simulink model "schemi_simulink"  (R2020a)
settings: Solver=VariableStepAuto  StartTime=0.0  StopTime=30  RelTol=1e-3
values from neighbouring files (symbols this model uses):
  A = [-m-a*y1/x_max+2*m*x1/x_max    a-a*x1/x_max;      b-b*y1/y_max  -n-b*x1/y_max+2*n*y1/y_max]    [linearized.m]
  A1 = [-m1-a1*y1/x_max1+2*m1*x1/x_max    a-a*x1/x_max1;      b1-b1*y1/y_max  -n1-b1*x1/y_max+2*n1*y1/y_max1]    [linearized.m]
  B = [1-x1/x_max;1-y1/y_max]    [linearized.m]
  B1 = [1-x1/x_max1;1-y1/y_max1]    [linearized.m]
  C = [1 0]    [linearized.m]
  D = 0    [linearized.m]
  dis = -0.3    [linearized.m]    (also in main.m = 0.3)
  Kf = KK(:,1:2)    [linearized.m]
  Kfm = KKm(:,1:2)    [linearized.m]
  Ki = KK(:,end)    [linearized.m]
  Kim = KKm(:,end)    [linearized.m]
  rif = 1    [linearized.m]    (also in main.m)
  td = 10    [linearized.m]
  x_ini = [0.1;0.1]    [linearized.m]
libraries: simulink x3
settings Model: Creator=ThinkPad  LastModifiedBy=ThinkPad

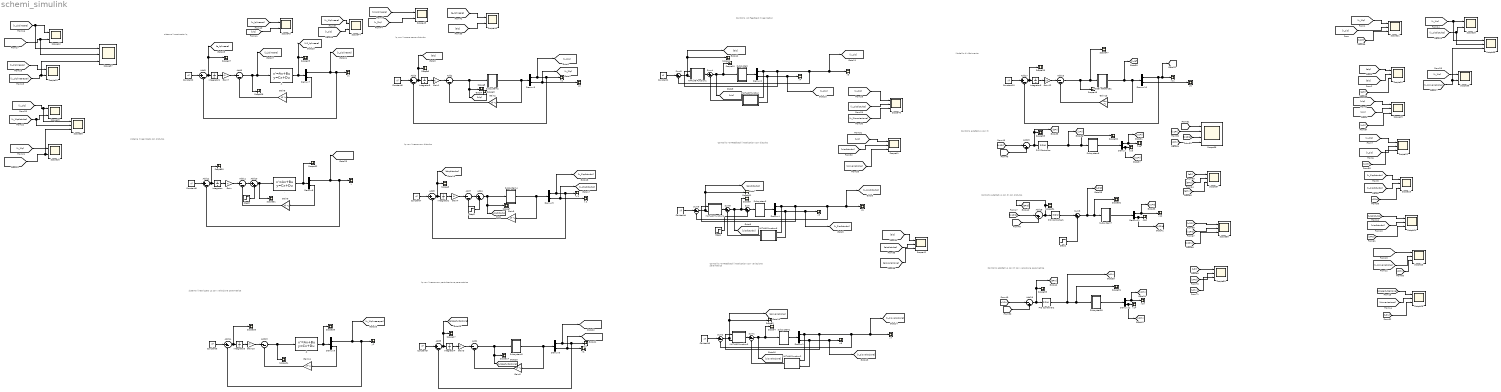
== system schemi_simulink ==
  note: Modello di riferimento
  note: Controllo I-O Feedback linearization
  note: Controllo I-O Feedback linearization con variazione parametrica
  note: Controllo I-O Feedback linearization con disturbo
  note: lq non lineare senza disturbo
  note: lq non lineare con disturbo
  note: lq non lineare con perturbazione parametrica
  note: sistema linearizzato lq
  note: sistema linearizzato con disturbo
  note: sistema linearizzato Lq con variazione parametrica
  note: Controllo adattativo con PI con disturbo
  note: Controllo adattativo con PI con variazione parametrica
  note: Controllo adattativo con PI
  . : StateSpace  A=A  B=B  C=[C; eye(2)]  D=[D; zeros(2,1)]  InitialCondition=x_ini
  .1 : StateSpace  A=A  B=B  C=[C; eye(2)]  D=[D; zeros(2,1)]  InitialCondition=x_ini
  .2 : StateSpace  A=A1  B=B1  C=[C; eye(2)]  D=[D; zeros(2,1)]  InitialCondition=x_ini
  Add{1..2,6..7,11,13,16} (7 alike) : Sum  Inputs=|--
  Add10 : Sum  Inputs=|++
  Add{3,5,8..9,12,14,17} (7 alike) : Sum  Inputs=|+-
  Add15 : Sum  Inputs=|-+
  Add18 : Sum  Inputs=|-+
  Add19 : Sum  Inputs=|-+
  Add4 : Sum  Inputs=|++
  Constant{1..10} (10 alike) : Constant  Value=rif
  Demux : Demux  Outputs=2
  Demux{1..6,10} (7 alike) : Demux  Outputs=[1 1]
  Demux11 : Demux  Outputs=2
  Demux12 : Demux  Outputs=2
  Demux7 : Demux  Outputs=[1 2]
  Demux8 : Demux  Outputs=[1 2]
  Demux9 : Demux  Outputs=[1 2]
  Gain{,1,3..4,7,10} (6 alike) : Gain  Gain=Ki
  Gain{2,5..6,8..9,11} (6 alike) : Gain  Gain=Kf  Multiplication=Matrix(K*u)
  Gain12 : Gain  Gain=Kim
  Gain13 : Gain  Gain=Kfm  Multiplication=Matrix(K*u)
  Integrator{,1..6} (7 alike) : Integrator
  MATLAB Function : MATLAB Function  TreatAsAtomicUnit=on
  MATLAB Function1 : MATLAB Function  TreatAsAtomicUnit=on
  MATLAB Function2 : MATLAB Function  TreatAsAtomicUnit=on
  MATLAB Function3 : MATLAB Function  TreatAsAtomicUnit=on
  MATLAB Function4 : MATLAB Function  TreatAsAtomicUnit=on
  MATLAB Function6 : MATLAB Function  TreatAsAtomicUnit=on
  Model reference1 : Subsystem
  PID Controller : simulink/Continuous/PID Controller  Controller=PID  Form=Parallel  TimeDomain=Continuous-time  UseExternalTs=off  SampleTime=-1  IntegratorMethod=Forward Euler  FilterMethod=Forward Euler  ControllerParametersSource=internal  P=10  I=20  D=0  UseFilter=on  N=100  TunerSelectOption=Transfer Function Based (PID Tuner App)  InitialConditionSource=internal  InitialConditionForIntegrator=0  InitialConditionForFilter=0  DifferentiatorICPrevScaledInput=0  ExternalReset=none  TrackingMode=off  Kt=1  LimitOutput=off  UpperSaturationLimit=inf  LowerSaturationLimit=-inf  LinearizeAsGain=on  AntiWindupMode=none  Kb=1  POutMin=[]  POutMax=[]  IOutMin=[]  IOutMax=[]  DOutMin=[]  DOutMax=[]  NOutMin=[]  NOutMax=[]  SumOutMin=[]  SumOutMax=[]  SaturationOutMin=[]  SaturationOutMax=[]  PParamMin=[]  PParamMax=[]  IParamMin=[]  IParamMax=[]  DParamMin=[]  DParamMax=[]  NParamMin=[]  NParamMax=[]  KbParamMin=[]  KbParamMax=[]  KtParamMin=[]  KtParamMax=[]  KbOutMin=[]  KbOutMax=[]  KtOutMin=[]  KtOutMax=[]  IntegratorOutMin=[]  IntegratorOutMax=[]  FilterOutMin=[]  FilterOutMax=[]  SumI1OutMin=[]  SumI1OutMax=[]  SumI2OutMin=[]  SumI2OutMax=[]  SumI3OutMin=[]  SumI3OutMax=[]  SumI4OutMin=[]  SumI4OutMax=[]  SumDOutMin=[]  SumDOutMax=[]  DifferentiatorOutMin=[]  DifferentiatorOutMax=[]  FilterDiffOutCoefMin=[]  FilterDiffOutCoefMax=[]  ReciprocalOutMin=[]  ReciprocalOutMax=[]  SumDenOutMin=[]  SumDenOutMax=[]  SumNumOutMin=[]  SumNumOutMax=[]  DivideOutMin=[]  DivideOutMax=[]  UdiffTsProdOutMin=[]  UdiffTsProdOutMax=[]  NTsProdOutMin=[]  NTsProdOutMax=[]  UintegralTsProdOutMin=[]  UintegralTsProdOutMax=[]  UngainTsProdOutMin=[]  UngainTsProdOutMax=[]  IntegratorContinuousStateAttributes=''  IntegratorStateMustResolveToSignalObject=off  IntegratorRTWStateStorageClass=Auto  FilterContinuousStateAttributes=''  FilterStateMustResolveToSignalObject=off  FilterRTWStateStorageClass=Auto  ParallelPVariant=InternalParameters  IdealPVariant=Disabled  IVariant=InternalParameters  DVariant=InternalParameters  IntegratorVariant=Continuous  SatVariant=Disabled  AWVariant=Passthrough  PCopyVariant=Disabled  TRVariant=Disabled  FdbkBlocksVariant=Forward  IdealPFdbkVariant=Disabled  SatFdbkVariant=Disabled  DerivativeFilterVariant=ContFilter  NVariant=InternalParameters  NCopyVariant=Disabled  FilterICVariant=InternalICsFilter  IntegratorICVariant=InternalICs  ExternalResetVariant=Disabled  TRSumVariant=Passthrough  SumFdbkVariant=Disabled  SumVariant=Sum_PID  TsampFilterVariant=InternalTs  TsampNgainVariant=Passthrough  TsampIntegralVariant=Passthrough
  PID Controller1 : simulink/Continuous/PID Controller  Controller=PID  Form=Parallel  TimeDomain=Continuous-time  UseExternalTs=off  SampleTime=-1  IntegratorMethod=Forward Euler  FilterMethod=Forward Euler  ControllerParametersSource=internal  P=10  I=20  D=0  UseFilter=on  N=100  TunerSelectOption=Transfer Function Based (PID Tuner App)  InitialConditionSource=internal  InitialConditionForIntegrator=0  InitialConditionForFilter=0  DifferentiatorICPrevScaledInput=0  ExternalReset=none  TrackingMode=off  Kt=1  LimitOutput=off  UpperSaturationLimit=inf  LowerSaturationLimit=-inf  LinearizeAsGain=on  AntiWindupMode=none  Kb=1  POutMin=[]  POutMax=[]  IOutMin=[]  IOutMax=[]  DOutMin=[]  DOutMax=[]  NOutMin=[]  NOutMax=[]  SumOutMin=[]  SumOutMax=[]  SaturationOutMin=[]  SaturationOutMax=[]  PParamMin=[]  PParamMax=[]  IParamMin=[]  IParamMax=[]  DParamMin=[]  DParamMax=[]  NParamMin=[]  NParamMax=[]  KbParamMin=[]  KbParamMax=[]  KtParamMin=[]  KtParamMax=[]  KbOutMin=[]  KbOutMax=[]  KtOutMin=[]  KtOutMax=[]  IntegratorOutMin=[]  IntegratorOutMax=[]  FilterOutMin=[]  FilterOutMax=[]  SumI1OutMin=[]  SumI1OutMax=[]  SumI2OutMin=[]  SumI2OutMax=[]  SumI3OutMin=[]  SumI3OutMax=[]  SumI4OutMin=[]  SumI4OutMax=[]  SumDOutMin=[]  SumDOutMax=[]  DifferentiatorOutMin=[]  DifferentiatorOutMax=[]  FilterDiffOutCoefMin=[]  FilterDiffOutCoefMax=[]  ReciprocalOutMin=[]  ReciprocalOutMax=[]  SumDenOutMin=[]  SumDenOutMax=[]  SumNumOutMin=[]  SumNumOutMax=[]  DivideOutMin=[]  DivideOutMax=[]  UdiffTsProdOutMin=[]  UdiffTsProdOutMax=[]  NTsProdOutMin=[]  NTsProdOutMax=[]  UintegralTsProdOutMin=[]  UintegralTsProdOutMax=[]  UngainTsProdOutMin=[]  UngainTsProdOutMax=[]  IntegratorContinuousStateAttributes=''  IntegratorStateMustResolveToSignalObject=off  IntegratorRTWStateStorageClass=Auto  FilterContinuousStateAttributes=''  FilterStateMustResolveToSignalObject=off  FilterRTWStateStorageClass=Auto  ParallelPVariant=InternalParameters  IdealPVariant=Disabled  IVariant=InternalParameters  DVariant=InternalParameters  IntegratorVariant=Continuous  SatVariant=Disabled  AWVariant=Passthrough  PCopyVariant=Disabled  TRVariant=Disabled  FdbkBlocksVariant=Forward  IdealPFdbkVariant=Disabled  SatFdbkVariant=Disabled  DerivativeFilterVariant=ContFilter  NVariant=InternalParameters  NCopyVariant=Disabled  FilterICVariant=InternalICsFilter  IntegratorICVariant=InternalICs  ExternalResetVariant=Disabled  TRSumVariant=Passthrough  SumFdbkVariant=Disabled  SumVariant=Sum_PID  TsampFilterVariant=InternalTs  TsampNgainVariant=Passthrough  TsampIntegralVariant=Passthrough
  PID Controller2 : simulink/Continuous/PID Controller  Controller=PID  Form=Parallel  TimeDomain=Continuous-time  UseExternalTs=off  SampleTime=-1  IntegratorMethod=Forward Euler  FilterMethod=Forward Euler  ControllerParametersSource=internal  P=10  I=20  D=0  UseFilter=on  N=100  TunerSelectOption=Transfer Function Based (PID Tuner App)  InitialConditionSource=internal  InitialConditionForIntegrator=0  InitialConditionForFilter=0  DifferentiatorICPrevScaledInput=0  ExternalReset=none  TrackingMode=off  Kt=1  LimitOutput=off  UpperSaturationLimit=inf  LowerSaturationLimit=-inf  LinearizeAsGain=on  AntiWindupMode=none  Kb=1  POutMin=[]  POutMax=[]  IOutMin=[]  IOutMax=[]  DOutMin=[]  DOutMax=[]  NOutMin=[]  NOutMax=[]  SumOutMin=[]  SumOutMax=[]  SaturationOutMin=[]  SaturationOutMax=[]  PParamMin=[]  PParamMax=[]  IParamMin=[]  IParamMax=[]  DParamMin=[]  DParamMax=[]  NParamMin=[]  NParamMax=[]  KbParamMin=[]  KbParamMax=[]  KtParamMin=[]  KtParamMax=[]  KbOutMin=[]  KbOutMax=[]  KtOutMin=[]  KtOutMax=[]  IntegratorOutMin=[]  IntegratorOutMax=[]  FilterOutMin=[]  FilterOutMax=[]  SumI1OutMin=[]  SumI1OutMax=[]  SumI2OutMin=[]  SumI2OutMax=[]  SumI3OutMin=[]  SumI3OutMax=[]  SumI4OutMin=[]  SumI4OutMax=[]  SumDOutMin=[]  SumDOutMax=[]  DifferentiatorOutMin=[]  DifferentiatorOutMax=[]  FilterDiffOutCoefMin=[]  FilterDiffOutCoefMax=[]  ReciprocalOutMin=[]  ReciprocalOutMax=[]  SumDenOutMin=[]  SumDenOutMax=[]  SumNumOutMin=[]  SumNumOutMax=[]  DivideOutMin=[]  DivideOutMax=[]  UdiffTsProdOutMin=[]  UdiffTsProdOutMax=[]  NTsProdOutMin=[]  NTsProdOutMax=[]  UintegralTsProdOutMin=[]  UintegralTsProdOutMax=[]  UngainTsProdOutMin=[]  UngainTsProdOutMax=[]  IntegratorContinuousStateAttributes=''  IntegratorStateMustResolveToSignalObject=off  IntegratorRTWStateStorageClass=Auto  FilterContinuousStateAttributes=''  FilterStateMustResolveToSignalObject=off  FilterRTWStateStorageClass=Auto  ParallelPVariant=InternalParameters  IdealPVariant=Disabled  IVariant=InternalParameters  DVariant=InternalParameters  IntegratorVariant=Continuous  SatVariant=Disabled  AWVariant=Passthrough  PCopyVariant=Disabled  TRVariant=Disabled  FdbkBlocksVariant=Forward  IdealPFdbkVariant=Disabled  SatFdbkVariant=Disabled  DerivativeFilterVariant=ContFilter  NVariant=InternalParameters  NCopyVariant=Disabled  FilterICVariant=InternalICsFilter  IntegratorICVariant=InternalICs  ExternalResetVariant=Disabled  TRSumVariant=Passthrough  SumFdbkVariant=Disabled  SumVariant=Sum_PID  TsampFilterVariant=InternalTs  TsampNgainVariant=Passthrough  TsampIntegralVariant=Passthrough
  Scope{1..11,14,17,27..35,47..55} (31 alike) : Scope
  Scope{12..13,15..16,18,36,43..46} (10 alike) : Scope  NumInputPorts=2
  Scope{19..26,37..42,57..59} (17 alike) : Scope  NumInputPorts=3
  Scope56 : Scope  NumInputPorts=4
  Step{1..2,5,8} (4 alike) : Step  Time=td  After=dis  SampleTime=0
  Subsystem : Subsystem
  Subsystem1 : Subsystem
  Subsystem2 : Subsystem
  Subsystem3 : Subsystem
  Subsystem4 : Subsystem
  Subsystem5 : Subsystem
  Subsystem6 : Subsystem
  Subsystem7 : Subsystem
  Subsystem9 : Subsystem
  Sum : Sum  Inputs=|++
  Sum{1..2,4..5,8..9} (6 alike) : Sum  Inputs=|+-
  Sum3 : Sum  Inputs=|++
  x.1 : Scope
  x.2 : Scope
  x{1..16} (16 alike) : Scope
  x1. : Scope
  x2. : Scope
  y : Scope
  y1 : Scope
  y2 : Scope
  wires:
  MATLAB Function/1(y) -> Sum4/2
  Constant1/1 -> Sum5/1
  Subsystem/1(Out1) -> Demux2/1
  MATLAB Function1/1(y) -> Sum4/1
  Sum5/1 -> [eio], Scope1/1, MATLAB Function1/2(e)  "e"
  Demux2/1 -> MATLAB Function/1(x_1), x3/1, [x_1io], Sum5/2, MATLAB Function1/1(x_1)
  Demux2/2 -> MATLAB Function/2(x_2), x4/1, [x_2io]
  Sum4/1 -> [uio], Scope10/1, Subsystem/1(u)  "u"
  Subsystem3/1(Out1) -> Demux4/1
  Demux4/2 -> MATLAB Function6/2(x_2), x5/1, [x_2iodisturbo]
  Demux4/1 -> MATLAB Function6/1(x_1), MATLAB Function4/1(x_1), x6/1, [x_1iodisturbo], Sum9/2
  Sum8/1 -> [uiodisturbo], Scope9/1, Sum/1  "u"
  Sum9/1 -> MATLAB Function4/2(e), Scope11/1, [eiodisturbo]  "e"
  Constant4/1 -> Sum9/1
  MATLAB Function4/1(y) -> Sum8/1
  MATLAB Function6/1(y) -> Sum8/2
  Sum/1 -> Subsystem3/1(u)
  Step1/1 -> Sum/2
  Subsystem1/1(Out1) -> Demux1/1
  Demux1/2 -> MATLAB Function2/2(x_2), x8/1, [x_2iovariazione]
  Demux1/1 -> MATLAB Function2/1(x_1), MATLAB Function3/1(x_1), x7/1, [x_1iovariazione], Sum2/2
  Sum1/1 -> [uiovariazione], Scope4/1, Subsystem1/1(u)  "u"
  Sum2/1 -> MATLAB Function3/2(e), Scope2/1, [eiovariazione]  "e"
  Constant3/1 -> Sum2/1
  MATLAB Function3/1(y) -> Sum1/1
  MATLAB Function2/1(y) -> Sum1/2
  Subsystem2/1(Out1) -> Gain2/1, Demux3/1
  Add2/1 -> [ulq], Scope5/1, Subsystem2/1(u)
  Integrator3/1 -> Gain1/1
  Constant5/1 -> Add3/1
  Demux3/2 -> x2/1, [x_2lq]
  Add3/1 -> Scope6/1, [elq], Integrator3/1
  Demux3/1 -> [x_1lq], x1/1, Add3/2
  Gain1/1 -> Add2/1
  Gain2/1 -> Add2/2
  Add8/1 -> Scope8/1, [elqdisturbo], Integrator2/1
  Constant7/1 -> Add8/1
  Add7/1 -> Add4/1
  Subsystem4/1(Out1) -> Gain5/1, Demux5/1
  Integrator2/1 -> Gain4/1
  Demux5/2 -> [x_2lqdisturbo], x.2/1
  Gain4/1 -> Add7/1
  Demux5/1 -> x.1/1, Add8/2, [x_1lqdisturbo]
  Add4/1 -> Subsystem4/1(u), [ulqdisturbo], Scope7/1
  Step5/1 -> Add4/2
  Gain5/1 -> Add7/2
  Add5/1 -> Scope17/1, [elqperturbazione], Integrator4/1
  Demux6/2 -> x2./1, [x_2lqperturbazione]
  Constant9/1 -> Add5/1
  Subsystem5/1(Out1) -> Gain6/1, Demux6/1
  Gain6/1 -> Add1/2
  Integrator4/1 -> Gain3/1
  Gain3/1 -> Add1/1
  Demux6/1 -> [x_1lqperturbazione], x1./1, Add5/2
  Add1/1 -> Scope14/1, [ulqperturbazione], Subsystem5/1(u)
  [x_1io] -> Scope21/2
  [elq] -> Scope20/1
  [eio] -> Scope20/2
  [ulq] -> Scope19/1
  [uio] -> Scope19/2
  [x_2lq] -> Scope22/1
  [x_2io] -> Scope22/2
  [x_1iodisturbo] -> Scope25/2
  [x_1lqdisturbo] -> Scope25/1
  [ulqdisturbo] -> Scope24/1
  [uiodisturbo] -> Scope24/2
  [uiovariazione] -> Scope26/2
  [ulqperturbazione] -> Scope26/1
  [x_1iovariazione] -> Scope23/2
  [x_1lqperturbazione] -> Scope23/1
  [x_1lq] -> Scope21/1
  Integrator1/1 -> Gain7/1
  Gain7/1 -> Add6/1
  Gain8/1 -> Add6/2
  Demux7/2 -> Gain8/1
  Demux7/1 -> [x_1lqlineare], y1/1, Add9/2
  .1/1 -> [x2_lqlineare], Scope29/1, Demux7/1
  Constant2/1 -> Add9/1
  Gain9/1 -> Add11/2
  Add12/1 -> Scope30/1, Integrator/1
  Gain/1 -> Add11/1
  Step8/1 -> Add10/2
  Add10/1 -> Scope31/1, ./1
  Demux8/2 -> Gain9/1
  Constant8/1 -> Add12/1
  Demux8/1 -> [x_1lqdisturbolineare], y/1, Add12/2
  ./1 -> Scope32/1, Demux8/1
  Integrator/1 -> Gain/1
  Add11/1 -> Add10/1
  Constant6/1 -> Add14/1
  .2/1 -> Scope35/1, Demux9/1
  Add13/1 -> Scope34/1, .2/1
  Demux9/1 -> [x_1lqlineareper], y2/1, Add14/2
  Demux9/2 -> Gain11/1
  Gain11/1 -> Add13/2
  Integrator5/1 -> Gain10/1
  Add14/1 -> Scope33/1, Integrator5/1
  Gain10/1 -> Add13/1
  [x_1lqlineare] -> Scope37/1, Scope12/1
  [x_1lqdisturbolineare] -> Scope37/2, Scope12/2
  [x_1lqlineare] -> Scope13/1
  [x_1lqlineareper] -> Scope37/3, Scope13/2
  [x_1lq] -> Scope38/1, Scope15/1
  [x_1lqdisturbo] -> Scope38/2, Scope15/2
  [x_1lq] -> Scope16/1
  [x_1lqperturbazione] -> Scope38/3, Scope16/2
  [x_1io] -> Scope39/1, Scope18/1
  [x_1iodisturbo] -> Scope39/2, Scope18/2
  [x_1io] -> Scope36/1
  [x_1iovariazione] -> Scope39/3, Scope36/2
  [x_2io] -> Scope40/1
  [x_2iodisturbo] -> Scope40/2
  [x_2iovariazione] -> Scope40/3
  [uio] -> Scope41/1
  [uiodisturbo] -> Scope41/2
  [uiovariazione] -> Scope41/3
  [eio] -> Scope42/1
  [eiodisturbo] -> Scope42/2
  [eiovariazione] -> Scope42/3
  Add6/1 -> Scope28/1, [u_lqlineare], .1/1
  Add9/1 -> [e_lqlineare], Scope27/1, Integrator1/1
  [u_lqlineare] -> Scope43/1
  [ulq] -> Scope43/2
  [x_1lqlineare] -> Scope44/1
  [x_1lq] -> Scope44/2
  [x2_lqlineare] -> Scope45/1
  [x_2lq] -> Scope45/2
  [e_lqlineare] -> Scope46/1
  [elq] -> Scope46/2
  [x1PI] -> Add15/1
  Subsystem6/1(Out1) -> Demux/1
  Add17/1 -> Scope49/1, Integrator6/1
  PID Controller/1 -> [uPI], Scope50/1, Subsystem6/1(u)
  Gain13/1 -> Add16/2
  Demux/2 -> [x2PI], x16/1
  Model reference1/1(Out1) -> [x_ref], Gain13/1, Demux10/1
  Demux10/2 -> x9/1
  Demux/1 -> x13/1, [x1PI]
  [x1_refPI] -> Add15/2
  Add16/1 -> Scope47/1, Model reference1/1(u), Scope48/1
  Demux10/1 -> x11/1, [x1_refPI], Add17/2
  Add15/1 -> [ePI], Scope53/1, PID Controller/1
  Constant10/1 -> Add17/1
  Integrator6/1 -> Gain12/1
  Gain12/1 -> Add16/1
  Add18/1 -> Scope54/1, [ePId], PID Controller1/1
  [x1_refPI] -> Add18/2
  Subsystem7/1(Out1) -> Demux11/1
  Demux11/1 -> [x1PId], x12/1
  [x1PId] -> Add18/1
  Step2/1 -> Sum3/2
  PID Controller1/1 -> Sum3/1
  Sum3/1 -> [uPId], Scope52/1, Subsystem7/1(u)
  Add19/1 -> [ePIv], Scope55/1, PID Controller2/1
  [x1_refPI] -> Add19/2
  Demux12/2 -> [x2PIv], x14/1
  Subsystem9/1(Out1) -> Demux12/1
  PID Controller2/1 -> [uPIv], Scope51/1, Subsystem9/1(u)
  Demux12/1 -> x10/1, [x1PIv]
  [x1PIv] -> Add19/1
  [x1_refPI] -> Scope56/1
  [x1PI] -> Scope56/2
  [x1PId] -> Scope56/3
  [x1PIv] -> Scope56/4
  [x1PI] -> Scope21/3
  [ePI] -> Scope20/3
  [uPI] -> Scope19/3
  [x2PI] -> Scope22/3
  [x1PIv] -> Scope23/3
  [x1PId] -> Scope25/3
  [uPId] -> Scope24/3
  [uPIv] -> Scope26/3
  Demux11/2 -> [x2PId], x15/1
  [ePI] -> Scope57/1
  [ePId] -> Scope57/2
  [ePIv] -> Scope57/3
  [x2PI] -> Scope58/1
  [x2PId] -> Scope58/2
  [x2PIv] -> Scope58/3
  [uPI] -> Scope59/1
  [uPId] -> Scope59/2
  [uPIv] -> Scope59/3

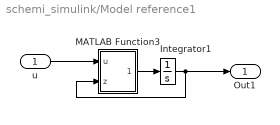
== system schemi_simulink/Model reference1 ==
  u : Inport
  Integrator1 : Integrator  InitialCondition=x_ini
  MATLAB Function3 : MATLAB Function  TreatAsAtomicUnit=on
  Out1 : Outport
  wires:
  u/1 -> MATLAB Function3/1(u)
  MATLAB Function3/1(xi_dot) -> Integrator1/1
  Integrator1/1 -> MATLAB Function3/2(z), Out1/1

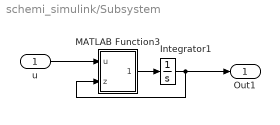
== system schemi_simulink/Subsystem ==
  u : Inport
  Integrator1 : Integrator  InitialCondition=x_ini
  MATLAB Function3 : MATLAB Function  TreatAsAtomicUnit=on
  Out1 : Outport
  wires:
  Integrator1/1 -> Out1/1, MATLAB Function3/2(z)
  MATLAB Function3/1(xi_dot) -> Integrator1/1
  u/1 -> MATLAB Function3/1(u)

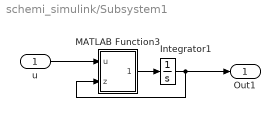
== system schemi_simulink/Subsystem1 ==
  u : Inport
  Integrator1 : Integrator  InitialCondition=x_ini
  MATLAB Function3 : MATLAB Function  TreatAsAtomicUnit=on
  Out1 : Outport
  wires:
  Integrator1/1 -> Out1/1, MATLAB Function3/2(z)
  MATLAB Function3/1(xi_dot) -> Integrator1/1
  u/1 -> MATLAB Function3/1(u)

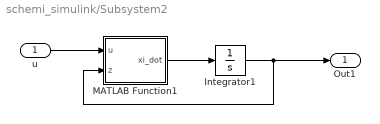
== system schemi_simulink/Subsystem2 ==
  u : Inport
  Integrator1 : Integrator  InitialCondition=x_ini
  MATLAB Function1 : MATLAB Function  TreatAsAtomicUnit=on
  Out1 : Outport
  wires:
  Integrator1/1 -> Out1/1, MATLAB Function1/2(z)
  MATLAB Function1/1(xi_dot) -> Integrator1/1
  u/1 -> MATLAB Function1/1(u)

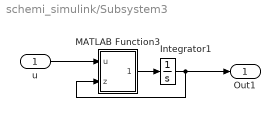
== system schemi_simulink/Subsystem3 ==
  u : Inport
  Integrator1 : Integrator  InitialCondition=x_ini
  MATLAB Function3 : MATLAB Function  TreatAsAtomicUnit=on
  Out1 : Outport
  wires:
  Integrator1/1 -> Out1/1, MATLAB Function3/2(z)
  MATLAB Function3/1(xi_dot) -> Integrator1/1
  u/1 -> MATLAB Function3/1(u)

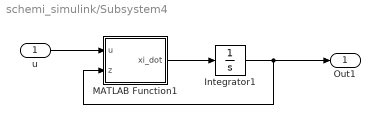
== system schemi_simulink/Subsystem4 ==
  u : Inport
  Integrator1 : Integrator  InitialCondition=x_ini
  MATLAB Function1 : MATLAB Function  TreatAsAtomicUnit=on
  Out1 : Outport
  wires:
  Integrator1/1 -> Out1/1, MATLAB Function1/2(z)
  MATLAB Function1/1(xi_dot) -> Integrator1/1
  u/1 -> MATLAB Function1/1(u)

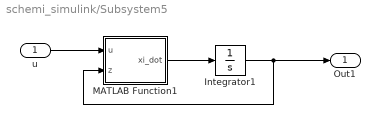
== system schemi_simulink/Subsystem5 ==
  u : Inport
  Integrator1 : Integrator  InitialCondition=x_ini
  MATLAB Function1 : MATLAB Function  TreatAsAtomicUnit=on
  Out1 : Outport
  wires:
  Integrator1/1 -> Out1/1, MATLAB Function1/2(z)
  MATLAB Function1/1(xi_dot) -> Integrator1/1
  u/1 -> MATLAB Function1/1(u)

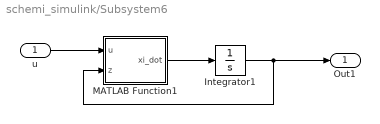
== system schemi_simulink/Subsystem6 ==
  u : Inport
  Integrator1 : Integrator  InitialCondition=x_ini
  MATLAB Function1 : MATLAB Function  TreatAsAtomicUnit=on
  Out1 : Outport
  wires:
  Integrator1/1 -> Out1/1, MATLAB Function1/2(z)
  MATLAB Function1/1(xi_dot) -> Integrator1/1
  u/1 -> MATLAB Function1/1(u)

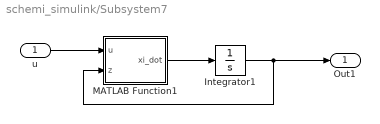
== system schemi_simulink/Subsystem7 ==
  u : Inport
  Integrator1 : Integrator  InitialCondition=x_ini
  MATLAB Function1 : MATLAB Function  TreatAsAtomicUnit=on
  Out1 : Outport
  wires:
  Integrator1/1 -> Out1/1, MATLAB Function1/2(z)
  MATLAB Function1/1(xi_dot) -> Integrator1/1
  u/1 -> MATLAB Function1/1(u)

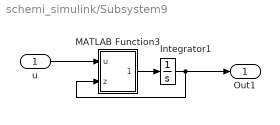
== system schemi_simulink/Subsystem9 ==
  u : Inport
  Integrator1 : Integrator  InitialCondition=x_ini
  MATLAB Function3 : MATLAB Function  TreatAsAtomicUnit=on
  Out1 : Outport
  wires:
  Integrator1/1 -> Out1/1, MATLAB Function3/2(z)
  MATLAB Function3/1(xi_dot) -> Integrator1/1
  u/1 -> MATLAB Function3/1(u)

== matlab function schemi_simulink/MATLAB Function4 ==
  data: x_1 input; y output; e input
function y = fcn2(x_1,e)
x1_max=5    
y=x1_max/(x1_max-x_1)*e;

== matlab function schemi_simulink/Subsystem7/MATLAB Function1 ==
  data: u input; xi_dot output; z input
function xi_dot = modello_fun(u,z)


a=1
b=2%
m=0.5
n=0.2
x_1_max=5
x_2_max=10



    xi_dot = [(1-z(1)/x_1_max)*(a*z(2)-m*z(1)+u);...
       (1-z(2)/x_2_max)*(b*z(1)-n*z(2)+u)];

end

== matlab function schemi_simulink/Subsystem9/MATLAB Function3 ==
  data: u input; xi_dot output; z input
function xi_dot = guerra_fun(u,z)%z tiene sia x che y
    %%inizializzazione

a=1
b=2
m=0.5
n=0.2
x_max=5
y_max=10
a1=a+10/100*a
b1=b+10/100*b
m1=m+10/100*m
n1=n+10/100*n
x_max1=x_max+10/100*x_max
y_max1=x_max+10/100*x_max


    xi_dot = [(1-z(1)/x_max1)*(a1*z(2)-m1*z(1)+u);...
       (1-z(2)/y_max1)*(b1*z(1)-n1*z(2)+u)];


end

== matlab function schemi_simulink/Model reference1/MATLAB Function3 ==
  data: u input; xi_dot output; z input
function xi_dot = guerra_fun(u,z)%z tiene sia x che y
    %%inizializzazione
% a=1
% b=2
% m=0.5
% n=0.2
% x_max=5
% y_max=10
% u=0
% 
% An=[-m -a; -b -n]
Am=[-0.5 0; 0 -0.2]
Bn=[1;1]
xi_dot=Am*z+Bn*u

end

== matlab function schemi_simulink/MATLAB Function ==
  data: x_1 input; y output; x_2 input
function y = fcn1(x_1,x_2)
a=1
b=2
m=0.5
n=0.2
x_1max=5
x_2max=10
y=-x_1max/(x_1max-x_1)*(-a*x_2+m*x_1+a/x_1max*x_1*x_2-m*x_1^2/x_1max);

== matlab function schemi_simulink/MATLAB Function2 ==
  data: x_1 input; y output; x_2 input
function y = fcn1(x_1,x_2)
a=1
b=2
m=0.5
n=0.2
x_1max=5
x_2max=10
y=-x_1max/(x_1max-x_1)*(-a*x_2+m*x_1+a/x_1max*x_1*x_2-m*x_1^2/x_1max);

== matlab function schemi_simulink/MATLAB Function3 ==
  data: x_1 input; y output; e input
function y = fcn2(x_1,e)
x1_max=5    
y=x1_max/(x1_max-x_1)*e;

== matlab function schemi_simulink/Subsystem/MATLAB Function3 ==
  data: u input; xi_dot output; z input
function xi_dot = guerra_fun(u,z)%z tiene sia x che y
    %%inizializzazione

a=1
b=2
%b=2.2/5
m=0.5
n=0.2
x_max=5
y_max=10
% x=4.9
% y=9.9
    xi_dot = [(1-z(1)/x_max)*(a*z(2)-m*z(1)+u);...
       (1-z(2)/y_max)*(b*z(1)-n*z(2)+u)];
% J1=[-m-a*y/x_max+2*m*x/x_max    a-a*x/x_max;...
%      b-b*y/y_max  -n-b*x/y_max+2*n*y/y_max];
end

== matlab function schemi_simulink/Subsystem1/MATLAB Function3 ==
  data: u input; xi_dot output; z input
function xi_dot = guerra_fun(u,z)%z tiene sia x che y
    %%inizializzazione

a=1
b=2
m=0.5
n=0.2
x_max=5
y_max=10
a1=a+10/100*a
b1=b+10/100*b
m1=m+10/100*m
n1=n+10/100*n
x_max1=x_max+10/100*x_max
y_max1=x_max+10/100*x_max


    xi_dot = [(1-z(1)/x_max1)*(a1*z(2)-m1*z(1)+u);...
       (1-z(2)/y_max1)*(b1*z(1)-n1*z(2)+u)];


end

== matlab function schemi_simulink/Subsystem2/MATLAB Function1 ==
  data: u input; xi_dot output; z input
function xi_dot = modello_fun(u,z)


a=1
b=2%
m=0.5
n=0.2
x_1_max=5
x_2_max=10



    xi_dot = [(1-z(1)/x_1_max)*(a*z(2)-m*z(1)+u);...
       (1-z(2)/x_2_max)*(b*z(1)-n*z(2)+u)];

end

== matlab function schemi_simulink/Subsystem4/MATLAB Function1 ==
  data: u input; xi_dot output; z input
function xi_dot = guerra_fun(u,z)%z tiene sia x che y
    %%inizializzazione

a=1
b=2%b=2.2/5
m=0.5
n=0.2
x_1_max=5
x_2_max=10



    xi_dot = [(1-z(1)/x_1_max)*(a*z(2)-m*z(1)+u);...
       (1-z(2)/x_2_max)*(b*z(1)-n*z(2)+u)];

end

== matlab function schemi_simulink/Subsystem5/MATLAB Function1 ==
  data: u input; xi_dot output; z input
function xi_dot = guerra_fun(u,z)%z tiene sia x che y
    %%inizializzazione

a=1
b=2
m=0.5
n=0.2
x_max=5
y_max=10
a1=a+10/100*a
b1=b+10/100*b
m1=m+10/100*m
n1=n+10/100*n
x_max1=x_max+10/100*x_max
y_max1=x_max+10/100*x_max


    xi_dot = [(1-z(1)/x_max1)*(a1*z(2)-m1*z(1)+u);...
       (1-z(2)/y_max1)*(b1*z(1)-n1*z(2)+u)];


end

== matlab function schemi_simulink/MATLAB Function1 ==
  data: x_1 input; y output; e input
function y = fcn2(x_1,e)
x1_max=5    
y=x1_max/(x1_max-x_1)*e;

== matlab function schemi_simulink/MATLAB Function6 ==
  data: x_1 input; y output; x_2 input
function y = fcn1(x_1,x_2)
a=1
b=2
m=0.5
n=0.2
x_1max=5
x_2max=10
y=-x_1max/(x_1max-x_1)*(-a*x_2+m*x_1+a/x_1max*x_1*x_2-m*x_1^2/x_1max);

== matlab function schemi_simulink/Subsystem6/MATLAB Function1 ==
  data: u input; xi_dot output; z input
function xi_dot = modello_fun(u,z)


a=1
b=2%
m=0.5
n=0.2
x_1_max=5
x_2_max=10



    xi_dot = [(1-z(1)/x_1_max)*(a*z(2)-m*z(1)+u);...
       (1-z(2)/x_2_max)*(b*z(1)-n*z(2)+u)];

end

== matlab function schemi_simulink/Subsystem3/MATLAB Function3 ==
  data: u input; xi_dot output; z input
function xi_dot = guerra_fun(u,z)%z tiene sia x che y
    %%inizializzazione

a=1
b=2
%b=2.2/5
m=0.5
n=0.2
x_max=5
y_max=10
% x=4.9
% y=9.9
    xi_dot = [(1-z(1)/x_max)*(a*z(2)-m*z(1)+u);...
       (1-z(2)/y_max)*(b*z(1)-n*z(2)+u)];
% J1=[-m-a*y/x_max+2*m*x/x_max    a-a*x/x_max;...
%      b-b*y/y_max  -n-b*x/y_max+2*n*y/y_max];
end
